simulink model "sim1"  (R2024a)
settings: Solver=FixedStepAuto  StartTime=0.0  StopTime=10.0  FixedStep=1e-3  RelTol=1e-3
libraries: simulink x3, matrix_library x1
settings Model: Creator=alexe  LastModifiedBy=alexe

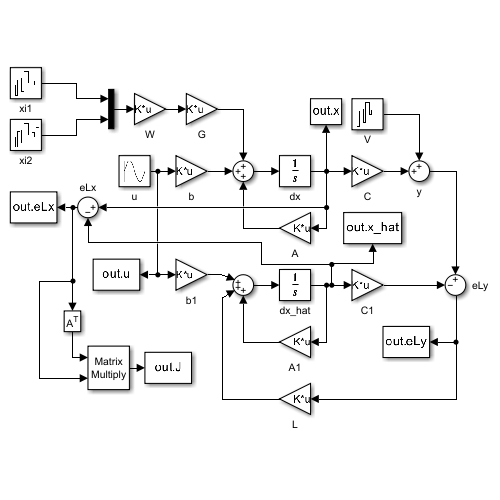
[thumbnail: Simulink's stored preview of the top-level diagram]
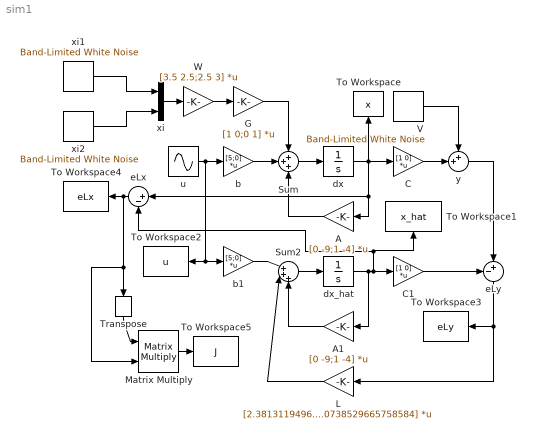
== system sim1 ==
  A : Gain  Gain=[0 -9;1 -4]  Multiplication=Matrix(K*u)
  A1 : Gain  Gain=[0 -9;1 -4]  Multiplication=Matrix(K*u)
  C : Gain  Gain=[1 0]  Multiplication=Matrix(K*u)
  C1 : Gain  Gain=[1 0]  Multiplication=Matrix(K*u)
  G : Gain  Gain=[1 0;0 1]  Multiplication=Matrix(K*u)
  L : Gain  Gain=[2.38131194966862;0.0738529665758584]  Multiplication=Matrix(K*u)
  Matrix Multiply : Product  Multiplication=Matrix(*)
  Sum : Sum  Inputs=+++
  Sum2 : Sum  Inputs=|+++
  To Workspace : ToWorkspace  VariableName=x  SaveFormat=Structure With Time  SampleTime=-1
  To Workspace1 : ToWorkspace  VariableName=x_hat  SaveFormat=Structure With Time  SampleTime=-1
  To Workspace2 : ToWorkspace  VariableName=u  SaveFormat=Structure With Time  SampleTime=-1
  To Workspace3 : ToWorkspace  VariableName=eLy  SaveFormat=Structure With Time  SampleTime=-1
  To Workspace4 : ToWorkspace  VariableName=eLx  SaveFormat=Structure With Time  SampleTime=-1
  To Workspace5 : ToWorkspace  VariableName=J  SaveFormat=Structure With Time  SampleTime=-1
  Transpose : matrix_library/Transpose
  V : simulink/Sources/Band-Limited White Noise  Cov=0.5  Ts=1e-3  seed=[3421]
  W : Gain  Gain=[3.5 2.5;2.5 3]  Multiplication=Matrix(K*u)
  b : Gain  Gain=[5;0]  Multiplication=Matrix(K*u)
  b1 : Gain  Gain=[5;0]  Multiplication=Matrix(K*u)
  dx : Integrator  InitialCondition=[1;0];
  dx_hat : Integrator  InitialCondition=[0;0];
  eLx : Sum  Inputs=|+-
  eLy : Sum  Inputs=-+|
  u : Sin  SampleTime=0
  xi : Mux  Inputs=2
  xi1 : simulink/Sources/Band-Limited White Noise  Cov=[1]  Ts=1e-3  seed=[1223]
  xi2 : simulink/Sources/Band-Limited White Noise  Cov=[1]  Ts=1e-3  seed=[23341]
  y : Sum  Inputs=++|
  wires:
  Sum/1 -> dx/1
  dx/1 -> To Workspace/1, C/1, eLx/1, A/1
  u/1 -> To Workspace2/1, b1/1, b/1
  C/1 -> y/2
  V/1 -> y/1
  b/1 -> Sum/2
  A/1 -> Sum/3
  Sum2/1 -> dx_hat/1
  dx_hat/1 -> C1/1, eLx/2, To Workspace1/1, A1/1
  b1/1 -> Sum2/1
  A1/1 -> Sum2/3
  C1/1 -> eLy/1
  y/1 -> eLy/2
  eLy/1 -> To Workspace3/1, L/1
  L/1 -> Sum2/2
  xi1/1 -> xi/1
  xi2/1 -> xi/2
  xi/1 -> W/1
  W/1 -> G/1
  eLx/1 -> Matrix Multiply/2, Transpose/1, To Workspace4/1
  Transpose/1 -> Matrix Multiply/1
  Matrix Multiply/1 -> To Workspace5/1
  G/1 -> Sum/1
